simulink model "HybridControllerD2D2withRot"  (R2015b)
settings: Solver=FixedStepDiscrete  SolverMode=SingleTasking  StartTime=0.0  StopTime=inf  FixedStep=controlPeriod  RelTol=1e-3
PreLoadFcn:
  | initializeSimulation
  | initializeSCRAMNetGT
  | ATS_setup_withRot
values from neighbouring files (symbols this model uses):
  controlPeriod = 1/2048    (= 0.00048828125)    [initializeSCRAMNetGT.m]
  MRC = [2 0.05 0.001]    [ATS_setup.m]
  nAcc = 11    [initializeSCRAMNetGT.m]
  nAct = 12    [initializeSCRAMNetGT.m]
  nAdcU = 40    [initializeSCRAMNetGT.m]
  nDucU = 4    [initializeSCRAMNetGT.m]
  Nl = floor(tl*sample_rate)    [ATS_setup.m]
  node = scgtnodestruct(node)    [initializeSCRAMNetGT.m]
  nTbl = 6    [initializeSCRAMNetGT.m]
  P_range = [0.7 1.30 ... (first row only)    [ATS_setup.m]
  sample = 1/2048    (= 0.00048828125)    [ATS_setup.m]
  SN = 16    [ATS_setup.m]
  Zden = ztag.Denominator{1}    [ATS_setup.m]
  Zden_Frc = ztag_Frc.Denominator{1}    [ATS_setup.m]
  Znum = ztag.Numerator{1}    [ATS_setup.m]
  Znum_Frc = ztag_Frc.Numerator{1}    [ATS_setup.m]
undefined symbols (not defined in the file or in its folder): msc150checks
undefined symbols (not defined in the file): HybridCtrlParameters, Par, Threshold
libraries: simulink x14, slrtlib x12, cwcec_scgtLib x4
(part 1 of 2)
CloseFcn:
  | rtwprivate ssgencode ModelCloseRequest scrnet_receiver
settings Model: ExtModeArmWhenConnect=off  Creator=aschellenberg  LastModifiedBy=Andreas
settings SolverCC: EnableConcurrentExecution=on
settings DataIOCC: LimitDataPoints=off  SaveFormat=Array  SaveOutput=off  SignalLogging=off  SaveTime=off  SignalLoggingName=sigsOut
settings OptimizationCC: BlockReduction=off  OptimizeBlockIOStorage=off  BufferReuse=off  GlobalBufferReuse=off  ExpressionFolding=off  ExpressionDepthLimit=2147483647  LocalBlockOutputs=off  InitFltsAndDblsToZero=on  EfficientFloat2IntCast=on  SimCompilerOptimization=on
settings DebuggingCC: SaveWithParameterizedLinksMsg=none  CheckSSInitialOutputMsg=off  UnderspecifiedInitializationDetection=Classic  MergeDetectMultiDrivingBlocksExec=none  StateNameClashWarn=warning
settings HardwareCC: ProdBitPerPointer=32  ProdLargestAtomicFloat=None  ProdWordSize=32  ProdLongLongMode=on  ProdHWDeviceType=Generic->32-bit x86 compatible  TargetHWDeviceType=32-bit Generic
settings SFSimCC: SimCustomHeaderCode="#include \"PredictorCorrector.h\""  SimUserSources=PredictorCorrector.c  SimUserIncludeDirs="\"C:\\Program Files\\OpenFresco\\SourceCode\\SRC\\experimentalControl\\Simulink\\HybridSimToolbox\""
settings RTWCC: SystemTargetFile=slrt.tlc  TemplateMakefile=slrt_default_tmf  Description=Simulink Real-Time  CustomHeaderCode="#include \"PredictorCorrector.h\""  CustomInclude="\"C:\\Program Files\\OpenFresco\\SourceCode\\SRC\\experimentalControl\\Simulink\\HybridSimToolbox\""  CustomSource=PredictorCorrector.c  RTWCompilerOptimization=on
settings SimulinkRealTimeCC: TargetFcnLib=ansi_tfl_tmw.mat  GeneratePreprocessorConditionals=Disable all  RL32IRQSourceModifier=Auto (PCI only)  xPCIRQSourceBoard=SCRAMNet_GT200
settings ConfigComp: CovModelRefEnable=Off  CovSFcnEnable=off

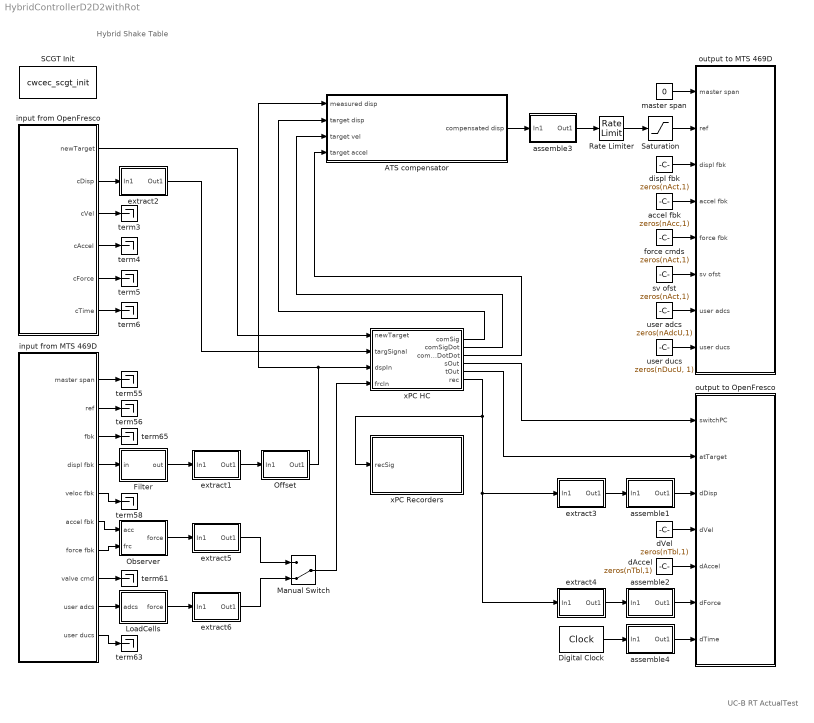
== system HybridControllerD2D2withRot ==
  note: Hybrid Shake Table
  note: UC-B RT ActualTest
  ATS compensator : Subsystem  mask{param=Par, threshold=Threshold}
      mask prompts: param "Initial a0, a1, a2 values :"; threshold "Threshold for triggering ATS :"
  Digital Clock : DigitalClock  SampleTime=controlPeriod
  Filter : Subsystem
  LoadCells : Subsystem
  Manual Switch : ManualSwitch  CurrentSetting=0
  Observer : Subsystem
  Offset : Subsystem  mask(Signal Offset){nS=HybridCtrlParameters.nDOF, nOffset=1}
      mask prompts: nS "Number of Signals: nS"; nOffset "Number of samples to initialize offset: nOffset"
      mask help:
      | Offset signal by average of signal over initial number of samples.
      | Set nOffset = -1 for no signal offset.
      mask Display: fprintf('Signal\nOffset')
  Rate Limiter : RateLimiter  RisingSlewLimit=[30 30 30 15 15 15]  FallingSlewLimit=-[30 30 30 15 15 15]  SampleTimeMode=inherited
  "SCGT Init " : S-Function  InitFcn=msc150checks(1)  FunctionName=cwcec_scgt_init  Parameters=node(1).Interface.Internal.NodeID, node(1).Interface.Internal.ActiveInterface, node.Interface.Internal.Options, node(1).Interface.Internal.Mask, pci  SFunctionDeploymentMode=off  EnableBusSupport=off  mask(SCGT Init){node=node, pci=-1}
      mask prompts: node "Node struct:"; pci "PCI slot (-1: autosearch):"
      mask help: Configures the SCRAMNet GT shared memory board. This is a required block for any model that uses shared memory with the SCRAMNet GT board. It configures important registers on the board acording to the user-defined node structure.
      mask init:
      | node=scgtnodestruct(node);
      mask Help: web([matlabroot '/toolbox/rtw/targets/xpc/target/build/xpcblocks/thirdpartydrivers/cwcec_scgthelp/'  'scgt5.html'])
      mask Display: disp('init')
  Saturation : Saturate  UpperLimit=[4.9 4.9 1.9 0.9 0.9 0.9]  LowerLimit=[-4.9 -4.9 -1.9 -0.9 -0.9 -0.9]
  accel fbk : Constant  Value=zeros(nAcc,1)
  assemble1 : Subsystem  mask(to Actuators){id=[1 2 3 4], size=nTbl}
      mask prompts: id "Index Vector: id"; size "Vector Size: size"
      mask help: To select to which actuator(s) the signals are going to
      mask Display: disp('Assemble')
  assemble2 : Subsystem  mask(to Actuators){id=[1 2 3 4], size=nTbl}
      mask prompts: id "Index Vector: id"; size "Vector Size: size"
      mask help: To select to which actuator(s) the signals are going to
      mask Display: disp('Assemble')
  assemble3 : Subsystem  mask(to Actuators){id=[1 2 4 5], size=nTbl}
      mask prompts: id "Index Vector: id"; size "Vector Size: size"
      mask help: To select to which actuator(s) the signals are going to
      mask Display: disp('Assemble')
  assemble4 : Subsystem  mask(to Actuators){id=1, size=nTbl}
      mask prompts: id "Index Vector: id"; size "Vector Size: size"
      mask help: To select to which actuator(s) the signals are going to
      mask Display: disp('Assemble')
  dAccel : Constant  Value=zeros(nTbl,1)
  dVel : Constant  Value=zeros(nTbl,1)
  displ fbk : Constant  Value=zeros(nAct,1)
  extract1 : Subsystem  mask(from Actuators){id=[1 2 4 5], size=5}
      mask prompts: id "Index Vector: id"; size "Vector Size: size"
      mask help: To select from which actuator(s) the signals are coming from
      mask Display: disp('Extract')
  extract2 : Subsystem  mask(from Actuators){id=[1 2 3 4], size=nTbl}
      mask prompts: id "Index Vector: id"; size "Vector Size: size"
      mask help: To select from which actuator(s) the signals are coming from
      mask Display: disp('Extract')
  extract3 : Subsystem  mask(from Actuators){id=[4*HybridCtrlParameters.nDOF+1:5*HybridCtrlParameters.nDOF], size=5+8*HybridCtrlParameters.nDOF}
      mask prompts: id "Index Vector: id"; size "Vector Size: size"
      mask help: To select from which actuator(s) the signals are coming from
      mask Display: disp('Extract')
  extract4 : Subsystem  mask(from Actuators){id=[5*HybridCtrlParameters.nDOF+1:6*HybridCtrlParameters.nDOF], size=5+8*HybridCtrlParameters.nDOF}
      mask prompts: id "Index Vector: id"; size "Vector Size: size"
      mask help: To select from which actuator(s) the signals are coming from
      mask Display: disp('Extract')
  extract5 : Subsystem  mask(from Actuators){id=[1 2 4 5], size=nTbl}
      mask prompts: id "Index Vector: id"; size "Vector Size: size"
      mask help: To select from which actuator(s) the signals are coming from
      mask Display: disp('Extract')
  extract6 : Subsystem  mask(from Actuators){id=[1 2 4 5], size=5}
      mask prompts: id "Index Vector: id"; size "Vector Size: size"
      mask help: To select from which actuator(s) the signals are coming from
      mask Display: disp('Extract')
  force cmds : Constant  Value=zeros(nAct,1)
  input from MTS 469D : Subsystem
  input from OpenFresco : Subsystem
  master span : Constant  Value=0
  output to MTS 469D : Subsystem
  output to OpenFresco : Subsystem
  sv ofst : Constant  Value=zeros(nAct,1)
  term{3..6,55..56,58,61,63,65} (10 alike) : Terminator
  user adcs : Constant  Value=zeros(nAdcU,1)
  user ducs : Constant  Value=zeros(nDucU, 1)  OutDataTypeStr=uint32
  xPC HC : Subsystem  mask(Hybrid Controller: D2/D2){nDOF=HybridCtrlParameters.nDOF, upFact=HybridCtrlParameters.upFact, dtInt=HybridCtrlParameters.dtInt, dtSim=HybridCtrlParameters.dtSim, dtCon=HybridCtrlParameters.dtCon, N=HybridCtrlParameters.N, iDelay=HybridCtrlParameters.iDelay}
      mask prompts: nDOF "Number of DOF: nDOF"; upFact "Upsample Factor: upFact"; dtInt "Integration time step: dtInt"; dtSim "Simulation time step: dtSim"; dtCon "Controller time step: dtCon"; N "Number of substeps: N"; iDelay "Number of delay steps: iDelay"
      mask help: Hybrid Controller using C0-continuous quadratic Lagrange interpolation for prediction and correction
      mask Display: disp('xPC Target\nHybrid Controller\n(D2/D2)')
  xPC Recorders : Subsystem  mask{nDOF=HybridCtrlParameters.nDOF}
      mask prompts: nDOF "Number of DOF: nDOF"
  wires:
  dVel/1 -> output to OpenFresco/4(dVel)
  dAccel/1 -> output to OpenFresco/5(dAccel)
  assemble4/1(Out1) -> output to OpenFresco/7(dTime)
  input from OpenFresco/3(cVel) -> term3/1
  input from OpenFresco/5(cForce) -> term5/1
  input from OpenFresco/6(cTime) -> term6/1
  assemble1/1(Out1) -> output to OpenFresco/3(dDisp)
  assemble2/1(Out1) -> output to OpenFresco/6(dForce)
  input from OpenFresco/2(cDisp) -> extract2/1(In1)
  input from OpenFresco/4(cAccel) -> term4/1
  input from OpenFresco/1(newTarget) -> xPC HC/1(newTarget)
  xPC HC/4(sOut) -> output to OpenFresco/1(switchPC)
  xPC HC/5(tOut) -> output to OpenFresco/2(atTarget)
  extract3/1(Out1) -> assemble1/1(In1)
  extract4/1(Out1) -> assemble2/1(In1)
  master span/1 -> output to MTS 469D/1(master span)
  force cmds/1 -> output to MTS 469D/5(force fbk)
  displ fbk/1 -> output to MTS 469D/3(displ fbk)
  user ducs/1 -> output to MTS 469D/8(user ducs)
  accel fbk/1 -> output to MTS 469D/4(accel fbk)
  user adcs/1 -> output to MTS 469D/7(user adcs)
  sv ofst/1 -> output to MTS 469D/6(sv ofst)
  Saturation/1 -> output to MTS 469D/2(ref)
  extract1/1(Out1) -> Offset/1(In1)
  input from MTS 469D/10(user ducs) -> term63/1
  input from MTS 469D/9(user adcs) -> LoadCells/1(adcs)
  input from MTS 469D/8(valve cmd) -> term61/1
  input from MTS 469D/7(force fbk) -> Observer/2(frc)
  input from MTS 469D/6(accel fbk) -> Observer/1(acc)
  input from MTS 469D/5(veloc fbk) -> term58/1
  input from MTS 469D/4(displ fbk) -> Filter/1(in)
  input from MTS 469D/2(ref) -> term56/1
  input from MTS 469D/1(master span) -> term55/1
  input from MTS 469D/3(fbk) -> term65/1
  Observer/1(force) -> extract5/1(In1)
  LoadCells/1(force) -> extract6/1(In1)
  xPC HC/6(rec) -> extract3/1(In1), extract4/1(In1), xPC Recorders/1(recSig)
  extract5/1(Out1) -> Manual Switch/1
  extract6/1(Out1) -> Manual Switch/2
  xPC HC/1(comSig) -> ATS compensator/2(target disp)
  xPC HC/2(comSigDot) -> ATS compensator/3(target vel)
  xPC HC/3(comSigDotDot) -> ATS compensator/4(target accel)
  Digital Clock/1 -> assemble4/1(In1)
  extract2/1(Out1) -> xPC HC/2(targSignal)
  Manual Switch/1 -> xPC HC/4(frcIn)
  Offset/1(Out1) -> ATS compensator/1(measured disp), xPC HC/3(dspIn)
  Filter/1(out) -> extract1/1(In1)
  Rate Limiter/1 -> Saturation/1
  ATS compensator/1(compensated disp) -> assemble3/1(In1)
  assemble3/1(Out1) -> Rate Limiter/1

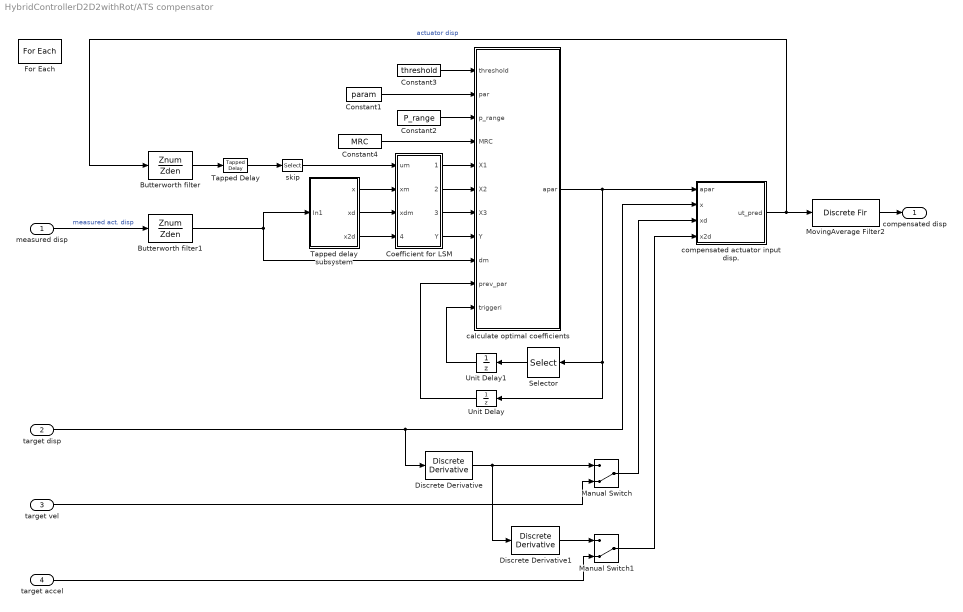
== system HybridControllerD2D2withRot/ATS compensator ==
  measured disp : Inport  Partition=on  PartitionDimension=1  PartitionWidth=1
  target disp : Inport  Port=2  Partition=on  PartitionDimension=1  PartitionWidth=1
  target vel : Inport  Port=3  Partition=on  PartitionDimension=1  PartitionWidth=1
  target accel : Inport  Port=4  Partition=on  PartitionDimension=1  PartitionWidth=1
  Butterworth filter : DiscreteTransferFcn  Numerator=Znum  Denominator=Zden  SampleTime=sample
  Butterworth filter1 : DiscreteTransferFcn  Numerator=Znum  Denominator=Zden  SampleTime=sample
  Coefficient for LSM : Subsystem
  Constant1 : Constant  Value=param
  Constant2 : Constant  Value=P_range
  Constant3 : Constant  Value=threshold
  Constant4 : Constant  Value=MRC
  Discrete Derivative : simulink/Discrete/Discrete Derivative  gainval=1.0  ICPrevScaledInput=0.0  OutMin=[]  OutMax=[]  OutDataType=fixdt(1, 16)  OutScaling=2^-10  DoSatur=off
  Discrete Derivative1 : simulink/Discrete/Discrete Derivative  gainval=1.0  ICPrevScaledInput=0.0  OutMin=[]  OutMax=[]  OutDataType=fixdt(1, 16)  OutScaling=2^-10  DoSatur=off
  For Each : ForEach  DisableCoverage=on  IterateSubsysMaskParameter=on,on  SubsysMaskParameterIterationDimension=2,2  IndexMode=One-based
  Manual Switch : ManualSwitch  CurrentSetting=0
  Manual Switch1 : ManualSwitch  CurrentSetting=0
  MovingAverage Filter2 : DiscreteFir  Coefficients=1/numSample*ones(1,numSample)  mask(Moving Average Filter){numSample=10}
      mask prompts: numSample "Number of Samples: numSample"
      mask help:
      | Moving average filter by using discrete FIR filter.
      | Set numSample = 1 for no filtering.
      mask Display: fprintf('MovingAverage\nFilter')
  Selector : Selector  InputPortWidth=4  IndexOptions=Index vector (dialog)  Indices=4  OutputSizes=1
  Tapped Delay : simulink/Discrete/Tapped Delay  vinit=0.0  samptime=-1  NumDelays=Nl  DelayOrder=Oldest  includeCurrent=off
  Tapped delay subsystem : Subsystem
  Unit Delay : UnitDelay  SampleTime=-1
  Unit Delay1 : UnitDelay  SampleTime=-1
  calculate optimal coefficients : MATLAB Function  TreatAsAtomicUnit=on
  compensated actuator input disp. : MATLAB Function  TreatAsAtomicUnit=on
  skip : Selector  InputPortWidth=Nl  IndexOptions=Index vector (dialog)  Indices=[1:SN:Nl]  OutputSizes=1
  compensated disp : Outport  ConcatenationDimension=1
  wires:
  measured disp/1 -> Butterworth filter1/1  "measured act. disp"
  Tapped Delay/1 -> skip/1
  calculate optimal coefficients/1(apar) -> Unit Delay/1, Selector/1, compensated actuator input disp./1(apar)
  compensated actuator input disp./1(ut_pred) -> MovingAverage Filter2/1, Butterworth filter/1  "actuator disp"
  Constant1/1 -> calculate optimal coefficients/2(par)
  Constant2/1 -> calculate optimal coefficients/3(p_range)
  Unit Delay/1 -> calculate optimal coefficients/10(prev_par)
  target disp/1 -> compensated actuator input disp./2(x), Discrete Derivative/1
  skip/1 -> Coefficient for LSM/1(um)
  Tapped delay subsystem/1(x) -> Coefficient for LSM/2(xm)
  Tapped delay subsystem/2(xd) -> Coefficient for LSM/3(xdm)
  Tapped delay subsystem/3(x2d) -> Coefficient for LSM/4(x2dm)
  Coefficient for LSM/1(X(1,:)) -> calculate optimal coefficients/5(X1)
  Coefficient for LSM/2(X(2,:)) -> calculate optimal coefficients/6(X2)
  Coefficient for LSM/3(X(3,:)) -> calculate optimal coefficients/7(X3)
  Coefficient for LSM/4(Y) -> calculate optimal coefficients/8(Y)
  Unit Delay1/1 -> calculate optimal coefficients/11(triggeri)
  Constant3/1 -> calculate optimal coefficients/1(threshold)
  Butterworth filter/1 -> Tapped Delay/1
  Constant4/1 -> calculate optimal coefficients/4(MRC)
  Selector/1 -> Unit Delay1/1
  Manual Switch/1 -> compensated actuator input disp./3(xd)
  Discrete Derivative/1 -> Manual Switch/1, Discrete Derivative1/1
  target vel/1 -> Manual Switch/2
  Discrete Derivative1/1 -> Manual Switch1/1
  Manual Switch1/1 -> compensated actuator input disp./4(x2d)
  target accel/1 -> Manual Switch1/2
  Butterworth filter1/1 -> Tapped delay subsystem/1(In1), calculate optimal coefficients/9(dm)
  MovingAverage Filter2/1 -> compensated disp/1

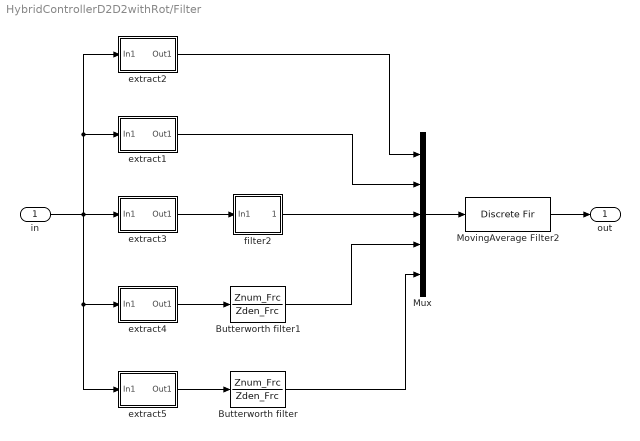
== system HybridControllerD2D2withRot/Filter ==
  in : Inport
  Butterworth filter : DiscreteTransferFcn  Numerator=Znum_Frc  Denominator=Zden_Frc  SampleTime=controlPeriod
  Butterworth filter1 : DiscreteTransferFcn  Numerator=Znum_Frc  Denominator=Zden_Frc  SampleTime=controlPeriod
  MovingAverage Filter2 : DiscreteFir  Coefficients=1/numSample*ones(1,numSample)  mask(Moving Average Filter){numSample=10}
      mask prompts: numSample "Number of Samples: numSample"
      mask help:
      | Moving average filter by using discrete FIR filter.
      | Set numSample = 1 for no filtering.
      mask Display: fprintf('MovingAverage\nFilter')
  Mux : Mux  Inputs=5
  extract1 : Subsystem  mask(from Actuators){id=2, size=nTbl}
      mask prompts: id "Index Vector: id"; size "Vector Size: size"
      mask help: To select from which actuator(s) the signals are coming from
      mask Display: disp('Extract')
  extract2 : Subsystem  mask(from Actuators){id=1, size=nTbl}
      mask prompts: id "Index Vector: id"; size "Vector Size: size"
      mask help: To select from which actuator(s) the signals are coming from
      mask Display: disp('Extract')
  extract3 : Subsystem  mask(from Actuators){id=3, size=nTbl}
      mask prompts: id "Index Vector: id"; size "Vector Size: size"
      mask help: To select from which actuator(s) the signals are coming from
      mask Display: disp('Extract')
  extract4 : Subsystem  mask(from Actuators){id=4, size=nTbl}
      mask prompts: id "Index Vector: id"; size "Vector Size: size"
      mask help: To select from which actuator(s) the signals are coming from
      mask Display: disp('Extract')
  extract5 : Subsystem  mask(from Actuators){id=5, size=nTbl}
      mask prompts: id "Index Vector: id"; size "Vector Size: size"
      mask help: To select from which actuator(s) the signals are coming from
      mask Display: disp('Extract')
  filter2 : Subsystem
  out : Outport
  wires:
  in/1 -> extract2/1(In1), extract1/1(In1), extract5/1(In1), extract4/1(In1), extract3/1(In1)
  Mux/1 -> MovingAverage Filter2/1
  extract1/1(Out1) -> Mux/2
  filter2/1(Out1) -> Mux/3
  extract3/1(Out1) -> filter2/1(In1)
  extract2/1(Out1) -> Mux/1
  extract4/1(Out1) -> Butterworth filter1/1
  MovingAverage Filter2/1 -> out/1
  extract5/1(Out1) -> Butterworth filter/1
  Butterworth filter/1 -> Mux/5
  Butterworth filter1/1 -> Mux/4

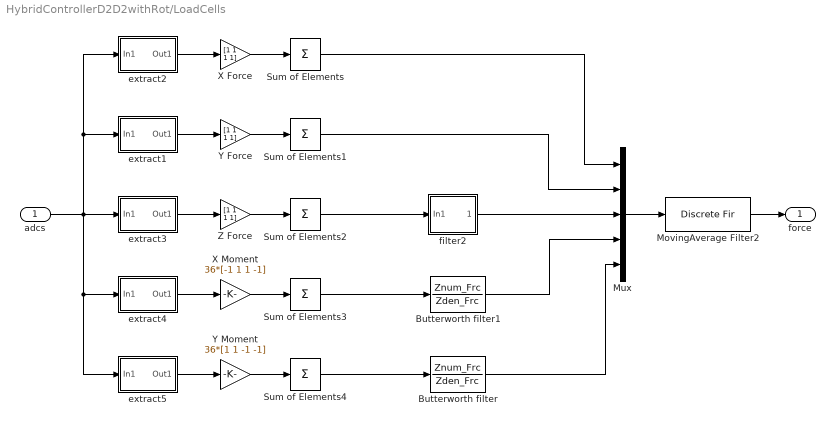
== system HybridControllerD2D2withRot/LoadCells ==
  adcs : Inport
  Butterworth filter : DiscreteTransferFcn  Numerator=Znum_Frc  Denominator=Zden_Frc  SampleTime=controlPeriod
  Butterworth filter1 : DiscreteTransferFcn  Numerator=Znum_Frc  Denominator=Zden_Frc  SampleTime=controlPeriod
  MovingAverage Filter2 : DiscreteFir  Coefficients=1/numSample*ones(1,numSample)  mask(Moving Average Filter){numSample=10}
      mask prompts: numSample "Number of Samples: numSample"
      mask help:
      | Moving average filter by using discrete FIR filter.
      | Set numSample = 1 for no filtering.
      mask Display: fprintf('MovingAverage\nFilter')
  Mux : Mux  Inputs=5
  Sum of Elements{,1..4} (5 alike) : Sum  Inputs=+
  X Force : Gain  Gain=[1 1 1 1]
  X Moment : Gain  Gain=36*[-1 1 1 -1]
  Y Force : Gain  Gain=[1 1 1 1]
  Y Moment : Gain  Gain=36*[1 1 -1 -1]
  Z Force : Gain  Gain=[1 1 1 1]
  extract1 : Subsystem  mask(from Actuators){id=[3 8 13 18], size=nAdcU}
      mask prompts: id "Index Vector: id"; size "Vector Size: size"
      mask help: To select from which actuator(s) the signals are coming from
      mask Display: disp('Extract')
  extract2 : Subsystem  mask(from Actuators){id=[2 7 12 17], size=nAdcU}
      mask prompts: id "Index Vector: id"; size "Vector Size: size"
      mask help: To select from which actuator(s) the signals are coming from
      mask Display: disp('Extract')
  extract3 : Subsystem  mask(from Actuators){id=[1 6 11 16], size=nAdcU}
      mask prompts: id "Index Vector: id"; size "Vector Size: size"
      mask help: To select from which actuator(s) the signals are coming from
      mask Display: disp('Extract')
  extract4 : Subsystem  mask(from Actuators){id=[1 6 11 16], size=nAdcU}
      mask prompts: id "Index Vector: id"; size "Vector Size: size"
      mask help: To select from which actuator(s) the signals are coming from
      mask Display: disp('Extract')
  extract5 : Subsystem  mask(from Actuators){id=[1 6 11 16], size=nAdcU}
      mask prompts: id "Index Vector: id"; size "Vector Size: size"
      mask help: To select from which actuator(s) the signals are coming from
      mask Display: disp('Extract')
  filter2 : Subsystem
  force : Outport
  wires:
  extract2/1(Out1) -> X Force/1
  adcs/1 -> extract2/1(In1), extract1/1(In1), extract5/1(In1), extract4/1(In1), extract3/1(In1)
  X Force/1 -> Sum of Elements/1
  extract1/1(Out1) -> Y Force/1
  Y Force/1 -> Sum of Elements1/1
  extract3/1(Out1) -> Z Force/1
  Z Force/1 -> Sum of Elements2/1
  Mux/1 -> MovingAverage Filter2/1
  Sum of Elements1/1 -> Mux/2
  Sum of Elements2/1 -> filter2/1(In1)
  filter2/1(Out1) -> Mux/3
  Sum of Elements/1 -> Mux/1
  extract4/1(Out1) -> X Moment/1
  X Moment/1 -> Sum of Elements3/1
  Sum of Elements3/1 -> Butterworth filter1/1
  extract5/1(Out1) -> Y Moment/1
  Y Moment/1 -> Sum of Elements4/1
  MovingAverage Filter2/1 -> force/1
  Sum of Elements4/1 -> Butterworth filter/1
  Butterworth filter/1 -> Mux/5
  Butterworth filter1/1 -> Mux/4

== system HybridControllerD2D2withRot/Observer ==
  acc : Inport
  frc : Inport  Port=2
  Add : Sum  Inputs=-+
  Mtable : Gain  Gain=[86.8 86.8 86.8 0.0 0.0 0.0]
  force : Outport
  wires:
  acc/1 -> Mtable/1
  Mtable/1 -> Add/1
  frc/1 -> Add/2
  Add/1 -> force/1

== system HybridControllerD2D2withRot/Offset ==
  In1 : Inport
  Constant : Constant  Value=zeros(1,nS)
  Counter : simulink/Sources/Counter Free-Running  NumBits=32  tsamp=controlPeriod
  Data Store Memory : DataStoreMemory  DataStoreName=x0  InitialValue=zeros(1,nS)  OutDataTypeStr=double
  Data Store Read : DataStoreRead  DataStoreName=x0  SampleTime=controlPeriod
  If : If  IfExpression=u1 < nOffset  ShowElse=off
  If Action : Subsystem  TreatAsAtomicUnit=on
  Sum1 : Sum  Inputs=+-|  SaturateOnIntegerOverflow=on  InputSameDT=on  OutDataTypeStr=Inherit: Same as first input
  Switch : Switch  Threshold=nOffset  SaturateOnIntegerOverflow=on  InputSameDT=on
  typeConv12 : DataTypeConversion  OutDataTypeStr=double  SaturateOnIntegerOverflow=on  RndMeth=Zero
  Out1 : Outport
  wires:
  Switch/1 -> Out1/1
  Sum1/1 -> Switch/1
  Data Store Read/1 -> Sum1/2
  In1/1 -> If Action/1(In1), Sum1/1
  Constant/1 -> Switch/3
  Counter/1 -> typeConv12/1
  If/1 -> If Action/Action
  typeConv12/1 -> Switch/2, If/1

== system HybridControllerD2D2withRot/assemble1 ==
  In1 : Inport
  Assignment : Assignment  OutputInitialize=Specify size for each dimension in table  IndexOptions=Index vector (port)  Indices=1  OutputSizes=size
  Constant : Constant  Value=id
  Out1 : Outport
  wires:
  Constant/1 -> Assignment/2
  Assignment/1 -> Out1/1
  In1/1 -> Assignment/1

== system HybridControllerD2D2withRot/assemble2 ==
  In1 : Inport
  Assignment : Assignment  OutputInitialize=Specify size for each dimension in table  IndexOptions=Index vector (port)  Indices=1  OutputSizes=size
  Constant : Constant  Value=id
  Out1 : Outport
  wires:
  Constant/1 -> Assignment/2
  Assignment/1 -> Out1/1
  In1/1 -> Assignment/1

== system HybridControllerD2D2withRot/assemble3 ==
  In1 : Inport
  Assignment : Assignment  OutputInitialize=Specify size for each dimension in table  IndexOptions=Index vector (port)  Indices=1  OutputSizes=size
  Constant : Constant  Value=id
  Out1 : Outport
  wires:
  Constant/1 -> Assignment/2
  Assignment/1 -> Out1/1
  In1/1 -> Assignment/1

== system HybridControllerD2D2withRot/assemble4 ==
  In1 : Inport
  Assignment : Assignment  OutputInitialize=Specify size for each dimension in table  IndexOptions=Index vector (port)  Indices=1  OutputSizes=size
  Constant : Constant  Value=id
  Out1 : Outport
  wires:
  Constant/1 -> Assignment/2
  Assignment/1 -> Out1/1
  In1/1 -> Assignment/1

== system HybridControllerD2D2withRot/extract1 ==
  In1 : Inport
  Selector : Selector  InputPortWidth=size  IndexOptions=Index vector (dialog)  Indices=id  OutputSizes=1
  Out1 : Outport
  wires:
  Selector/1 -> Out1/1
  In1/1 -> Selector/1

== system HybridControllerD2D2withRot/extract2 ==
  In1 : Inport
  Selector : Selector  InputPortWidth=size  IndexOptions=Index vector (dialog)  Indices=id  OutputSizes=1
  Out1 : Outport
  wires:
  Selector/1 -> Out1/1
  In1/1 -> Selector/1

== system HybridControllerD2D2withRot/extract3 ==
  In1 : Inport
  Selector : Selector  InputPortWidth=size  IndexOptions=Index vector (dialog)  Indices=id  OutputSizes=1
  Out1 : Outport
  wires:
  Selector/1 -> Out1/1
  In1/1 -> Selector/1

== system HybridControllerD2D2withRot/extract4 ==
  In1 : Inport
  Selector : Selector  InputPortWidth=size  IndexOptions=Index vector (dialog)  Indices=id  OutputSizes=1
  Out1 : Outport
  wires:
  Selector/1 -> Out1/1
  In1/1 -> Selector/1

== system HybridControllerD2D2withRot/extract5 ==
  In1 : Inport
  Selector : Selector  InputPortWidth=size  IndexOptions=Index vector (dialog)  Indices=id  OutputSizes=1
  Out1 : Outport
  wires:
  Selector/1 -> Out1/1
  In1/1 -> Selector/1

== system HybridControllerD2D2withRot/extract6 ==
  In1 : Inport
  Selector : Selector  InputPortWidth=size  IndexOptions=Index vector (dialog)  Indices=id  OutputSizes=1
  Out1 : Outport
  wires:
  Selector/1 -> Out1/1
  In1/1 -> Selector/1

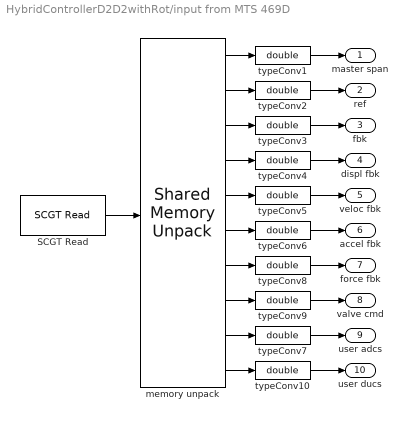
== system HybridControllerD2D2withRot/input from MTS 469D ==
  "SCGT Read " : cwcec_scgtLib/SCGT Read   partition=node.Partitions(9:18)  ts=controlPeriod  pci=-1
  memory unpack : slrtlib/Shared Memory/Shared Memory Unpack   partition=node.Partitions(9:18)
  typeConv{1..10} (10 alike) : DataTypeConversion  OutDataTypeStr=double  SaturateOnIntegerOverflow=on  RndMeth=Zero
  master span : Outport
  ref : Outport  Port=2
  fbk : Outport  Port=3
  displ fbk : Outport  Port=4
  veloc fbk : Outport  Port=5
  accel fbk : Outport  Port=6
  force fbk : Outport  Port=7
  valve cmd : Outport  Port=8
  user adcs : Outport  Port=9
  user ducs : Outport  Port=10
  wires:
  memory unpack/10 -> typeConv10/1
  memory unpack/9 -> typeConv7/1
  memory unpack/8 -> typeConv9/1
  memory unpack/7 -> typeConv8/1
  memory unpack/6 -> typeConv6/1
  memory unpack/5 -> typeConv5/1
  memory unpack/4 -> typeConv4/1
  memory unpack/3 -> typeConv3/1
  memory unpack/2 -> typeConv2/1
  memory unpack/1 -> typeConv1/1
  typeConv2/1 -> ref/1
  typeConv1/1 -> master span/1
  "SCGT Read "/1 -> memory unpack/1
  typeConv3/1 -> fbk/1
  typeConv4/1 -> displ fbk/1
  typeConv5/1 -> veloc fbk/1
  typeConv6/1 -> accel fbk/1
  typeConv8/1 -> force fbk/1
  typeConv9/1 -> valve cmd/1
  typeConv7/1 -> user adcs/1
  typeConv10/1 -> user ducs/1

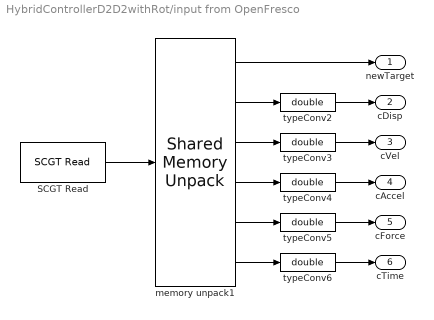
== system HybridControllerD2D2withRot/input from OpenFresco ==
  SCGT Read : cwcec_scgtLib/SCGT Read   partition=node.Partitions(19:24)  ts=controlPeriod  pci=-1
  memory unpack1 : slrtlib/Shared Memory/Shared Memory Unpack   partition=node.Partitions(19:24)
  typeConv{2..6} (5 alike) : DataTypeConversion  OutDataTypeStr=double  SaturateOnIntegerOverflow=on  RndMeth=Zero
  newTarget : Outport
  cDisp : Outport  Port=2
  cVel : Outport  Port=3
  cAccel : Outport  Port=4
  cForce : Outport  Port=5
  cTime : Outport  Port=6
  wires:
  typeConv2/1 -> cDisp/1
  typeConv3/1 -> cVel/1
  typeConv4/1 -> cAccel/1
  typeConv5/1 -> cForce/1
  typeConv6/1 -> cTime/1
  memory unpack1/3 -> typeConv3/1
  memory unpack1/4 -> typeConv4/1
  memory unpack1/6 -> typeConv6/1
  memory unpack1/5 -> typeConv5/1
  SCGT Read/1 -> memory unpack1/1
  memory unpack1/2 -> typeConv2/1
  memory unpack1/1 -> newTarget/1

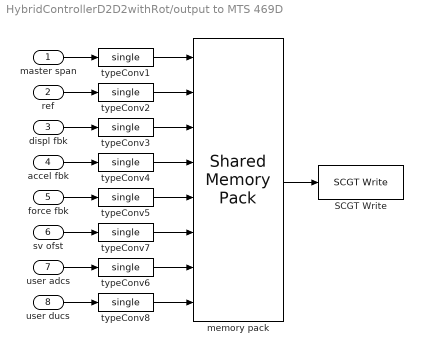
== system HybridControllerD2D2withRot/output to MTS 469D ==
  master span : Inport
  ref : Inport  Port=2
  displ fbk : Inport  Port=3
  accel fbk : Inport  Port=4
  force fbk : Inport  Port=5
  sv ofst : Inport  Port=6
  user adcs : Inport  Port=7
  user ducs : Inport  Port=8
  "SCGT Write " : cwcec_scgtLib/SCGT Write   partition=node.Partitions(1:8)  ts=controlPeriod  pci=-1
  memory pack : slrtlib/Shared Memory/Shared Memory Pack   partition=node.Partitions(1:8)
  typeConv{1..8} (8 alike) : DataTypeConversion  OutDataTypeStr=single  SaturateOnIntegerOverflow=on  RndMeth=Zero
  wires:
  typeConv8/1 -> memory pack/8
  user ducs/1 -> typeConv8/1
  user adcs/1 -> typeConv6/1
  sv ofst/1 -> typeConv7/1
  master span/1 -> typeConv1/1
  ref/1 -> typeConv2/1
  displ fbk/1 -> typeConv3/1
  accel fbk/1 -> typeConv4/1
  memory pack/1 -> "SCGT Write "/1
  typeConv1/1 -> memory pack/1
  typeConv2/1 -> memory pack/2
  typeConv3/1 -> memory pack/3
  typeConv4/1 -> memory pack/4
  force fbk/1 -> typeConv5/1
  typeConv5/1 -> memory pack/5
  typeConv7/1 -> memory pack/6
  typeConv6/1 -> memory pack/7

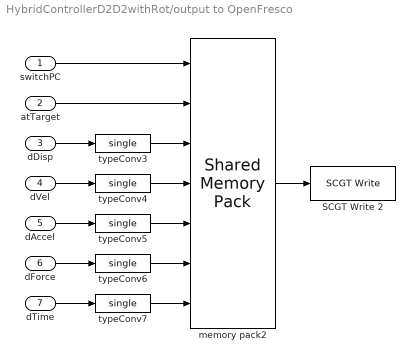
== system HybridControllerD2D2withRot/output to OpenFresco ==
  switchPC : Inport
  atTarget : Inport  Port=2
  dDisp : Inport  Port=3
  dVel : Inport  Port=4
  dAccel : Inport  Port=5
  dForce : Inport  Port=6
  dTime : Inport  Port=7
  SCGT Write 2 : cwcec_scgtLib/SCGT Write   partition=node.Partitions(25:31)  ts=controlPeriod  pci=-1
  memory pack2 : slrtlib/Shared Memory/Shared Memory Pack   partition=node.Partitions(25:31)
  typeConv{3..7} (5 alike) : DataTypeConversion  OutDataTypeStr=single  SaturateOnIntegerOverflow=on  RndMeth=Zero
  wires:
  dAccel/1 -> typeConv5/1
  dVel/1 -> typeConv4/1
  dDisp/1 -> typeConv3/1
  typeConv4/1 -> memory pack2/4
  typeConv5/1 -> memory pack2/5
  dForce/1 -> typeConv6/1
  typeConv6/1 -> memory pack2/6
  dTime/1 -> typeConv7/1
  typeConv7/1 -> memory pack2/7
  memory pack2/1 -> SCGT Write 2/1
  typeConv3/1 -> memory pack2/3
  atTarget/1 -> memory pack2/2
  switchPC/1 -> memory pack2/1

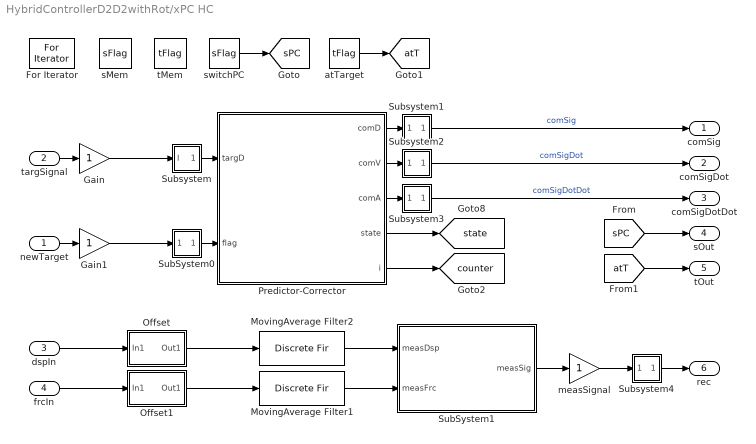
== system HybridControllerD2D2withRot/xPC HC ==
  newTarget : Inport
  targSignal : Inport  Port=2
  dspIn : Inport  Port=3
  frcIn : Inport  Port=4
  For Iterator : ForIterator  IterationLimit=upFact  ShowIterationPort=off
  Gain : Gain  OutDataTypeStr=double
  Gain1 : Gain  OutDataTypeStr=int32
  MovingAverage Filter1 : DiscreteFir  Coefficients=1/numSample*ones(1,numSample)  mask(Moving Average Filter){numSample=1}
      mask prompts: numSample "Number of Samples: numSample"
      mask help:
      | Moving average filter by using discrete FIR filter.
      | Set numSample = 1 for no filtering.
      mask Display: fprintf('MovingAverage\nFilter')
  MovingAverage Filter2 : DiscreteFir  Coefficients=1/numSample*ones(1,numSample)  mask(Moving Average Filter){numSample=1}
      mask prompts: numSample "Number of Samples: numSample"
      mask help:
      | Moving average filter by using discrete FIR filter.
      | Set numSample = 1 for no filtering.
      mask Display: fprintf('MovingAverage\nFilter')
  Offset : Subsystem  mask(Signal Offset){nS=nDOF, nOffset=1/dtCon}
      mask prompts: nS "Number of Signals: nS"; nOffset "Number of samples to initialize offset: nOffset"
      mask help:
      | Offset signal by average of signal over initial number of samples.
      | Set nOffset = -1 for no signal offset.
      mask Display: fprintf('Signal\nOffset')
  Offset1 : Subsystem  mask(Signal Offset){nS=nDOF, nOffset=1/dtCon}
      mask prompts: nS "Number of Signals: nS"; nOffset "Number of samples to initialize offset: nOffset"
      mask help:
      | Offset signal by average of signal over initial number of samples.
      | Set nOffset = -1 for no signal offset.
      mask Display: fprintf('Signal\nOffset')
  Predictor-Corrector : Stateflow chart  TreatAsAtomicUnit=on
  SubSystem0 : Subsystem
      mask Display: disp('I/O')
  SubSystem1 : Subsystem
  Subsystem : Subsystem
      mask Display: disp('I/O')
  Subsystem1 : Subsystem
      mask Display: disp('I/O')
  Subsystem2 : Subsystem
      mask Display: disp('I/O')
  Subsystem3 : Subsystem
      mask Display: disp('I/O')
  Subsystem4 : Subsystem
      mask Display: disp('I/O')
  atTarget : DataStoreRead  DataStoreName=tFlag
  measSignal : Gain  OutDataTypeStr=double
  sMem : DataStoreMemory  DataStoreName=sFlag  OutDataTypeStr=int32
  switchPC : DataStoreRead  DataStoreName=sFlag
  tMem : DataStoreMemory  DataStoreName=tFlag  OutDataTypeStr=int32
  comSig : Outport
  comSigDot : Outport  Port=2
  comSigDotDot : Outport  Port=3
  sOut : Outport  Port=4
  tOut : Outport  Port=5
  rec : Outport  Port=6
  tag scope: atT=global, counter=global, sPC=global, state=global
  wires:
  frcIn/1 -> Offset1/1(In1)
  measSignal/1 -> Subsystem4/1(measSig)
  dspIn/1 -> Offset/1(In1)
  SubSystem1/1(measSig) -> measSignal/1
  Predictor-Corrector/5(i) -> [counter]
  SubSystem0/1(Out) -> Predictor-Corrector/2(flag)
  newTarget/1 -> Gain1/1
  switchPC/1 -> [sPC]
  atTarget/1 -> [atT]
  targSignal/1 -> Gain/1
  Subsystem/1(O) -> Predictor-Corrector/1(targD)
  MovingAverage Filter2/1 -> SubSystem1/1(measDsp)
  MovingAverage Filter1/1 -> SubSystem1/2(measFrc)
  Predictor-Corrector/1(comD) -> Subsystem1/1(In)
  Predictor-Corrector/2(comV) -> Subsystem2/1(In)
  Predictor-Corrector/3(comA) -> Subsystem3/1(In)
  Gain/1 -> Subsystem/1(I)
  Gain1/1 -> SubSystem0/1(In)
  Offset/1(Out1) -> MovingAverage Filter2/1
  Predictor-Corrector/4(state) -> [state]
  Subsystem2/1(Out) -> comSigDot/1  "comSigDot"
  Subsystem3/1(Out) -> comSigDotDot/1  "comSigDotDot"
  Subsystem1/1(Out) -> comSig/1  "comSig"
  Subsystem4/1(Out1) -> rec/1
  [sPC] -> sOut/1
  [atT] -> tOut/1
  Offset1/1(Out1) -> MovingAverage Filter1/1

== system HybridControllerD2D2withRot/xPC Recorders ==
  recSig : Inport
  Demux : Demux  Outputs=[nDOF (3*nDOF) (2*nDOF) 1 1 3 nDOF nDOF]
  "Scope (xPC) " : slrtlib/Displays and Logging/Scope   scopeno=4  scopetype=File  autostart=on  viewmode=Graphical redraw  formatstr='%15.6f'  grid=on  ylimits=[0,3]  nosamples=60*2048  noprepostsamples=0  interleave=1  triggermode=FreeRun  triggersignal=1  trigsignalfromport=off  triggerlevel=0.0  triggerslope=Either  triggerscope=1  triggersample=0  filename=state.dat  mode=Lazy  writesize=512  autorestart=on  dynamicfilemode=off  maxwritefilesize=512*1024^2
  Scope (xPC) 1 : slrtlib/Displays and Logging/Scope   scopeno=1  scopetype=File  autostart=on  viewmode=Numerical  formatstr='%15.6f'  grid=on  ylimits=[-4,4]  nosamples=60*2048  noprepostsamples=0  interleave=1  triggermode=FreeRun  triggersignal=1  trigsignalfromport=off  triggerlevel=0.0  triggerslope=Either  triggerscope=1  triggersample=0  filename=targSig.dat  mode=Lazy  writesize=512  autorestart=on  dynamicfilemode=off  maxwritefilesize=512*1024^2
  Scope (xPC) 2 : slrtlib/Displays and Logging/Scope   scopeno=5  scopetype=File  autostart=on  viewmode=Numerical  formatstr='%15.6f'  grid=on  ylimits=[0,3]  nosamples=60*2048  noprepostsamples=0  interleave=1  triggermode=FreeRun  triggersignal=1  trigsignalfromport=off  triggerlevel=0.0  triggerslope=Either  triggerscope=1  triggersample=0  filename=count.dat  mode=Lazy  writesize=512  autorestart=on  dynamicfilemode=off  maxwritefilesize=512*1024^2
  Scope (xPC) 3 : slrtlib/Displays and Logging/Scope   scopeno=6  scopetype=File  autostart=on  viewmode=Numerical  formatstr='%15.6f'  grid=on  ylimits=[0,3]  nosamples=60*2048  noprepostsamples=0  interleave=1  triggermode=FreeRun  triggersignal=1  trigsignalfromport=off  triggerlevel=0.0  triggerslope=Either  triggerscope=1  triggersample=0  filename=flag.dat  mode=Lazy  writesize=512  autorestart=on  dynamicfilemode=off  maxwritefilesize=512*1024^2
  Scope (xPC) 4 : slrtlib/Displays and Logging/Scope   scopeno=2  scopetype=File  autostart=on  viewmode=Numerical  formatstr='%15.6f'  grid=on  ylimits=[-4,4]  nosamples=60*2048  noprepostsamples=0  interleave=1  triggermode=FreeRun  triggersignal=1  trigsignalfromport=off  triggerlevel=0.0  triggerslope=Either  triggerscope=1  triggersample=0  filename=commSig.dat  mode=Lazy  writesize=512  autorestart=on  dynamicfilemode=off  maxwritefilesize=512*1024^2
  Scope (xPC) 5 : slrtlib/Displays and Logging/Scope   scopeno=3  scopetype=File  autostart=on  viewmode=Numerical  formatstr='%15.6f'  grid=on  ylimits=[-4,4]  nosamples=60*2048  noprepostsamples=0  interleave=1  triggermode=FreeRun  triggersignal=1  trigsignalfromport=off  triggerlevel=0.0  triggerslope=Either  triggerscope=1  triggersample=0  filename=measSig.dat  mode=Lazy  writesize=512  autorestart=on  dynamicfilemode=off  maxwritefilesize=512*1024^2
  Scope (xPC) 6 : slrtlib/Displays and Logging/Scope   scopeno=7  scopetype=File  autostart=on  viewmode=Graphical redraw  formatstr='%15.6f'  grid=on  ylimits=[-1,1]  nosamples=60*2048  noprepostsamples=0  interleave=1  triggermode=FreeRun  triggersignal=1  trigsignalfromport=off  triggerlevel=0.0  triggerslope=Either  triggerscope=1  triggersample=0  filename=measDsp.dat  mode=Lazy  writesize=512  autorestart=on  dynamicfilemode=off  maxwritefilesize=512*1024^2
  Scope (xPC) 7 : slrtlib/Displays and Logging/Scope   scopeno=8  scopetype=File  autostart=on  viewmode=Numerical  formatstr='%15.6f'  grid=on  ylimits=[0,3]  nosamples=60*2048  noprepostsamples=0  interleave=1  triggermode=FreeRun  triggersignal=1  trigsignalfromport=off  triggerlevel=0.0  triggerslope=Either  triggerscope=1  triggersample=0  filename=measFrc.dat  mode=Lazy  writesize=512  autorestart=on  dynamicfilemode=off  maxwritefilesize=512*1024^2
  wires:
  recSig/1 -> Demux/1
  Demux/1 -> Scope (xPC) 1/1
  Demux/2 -> Scope (xPC) 4/1
  Demux/3 -> Scope (xPC) 5/1
  Demux/4 -> "Scope (xPC) "/1
  Demux/5 -> Scope (xPC) 2/1
  Demux/6 -> Scope (xPC) 3/1
  Demux/8 -> Scope (xPC) 7/1
  Demux/7 -> Scope (xPC) 6/1

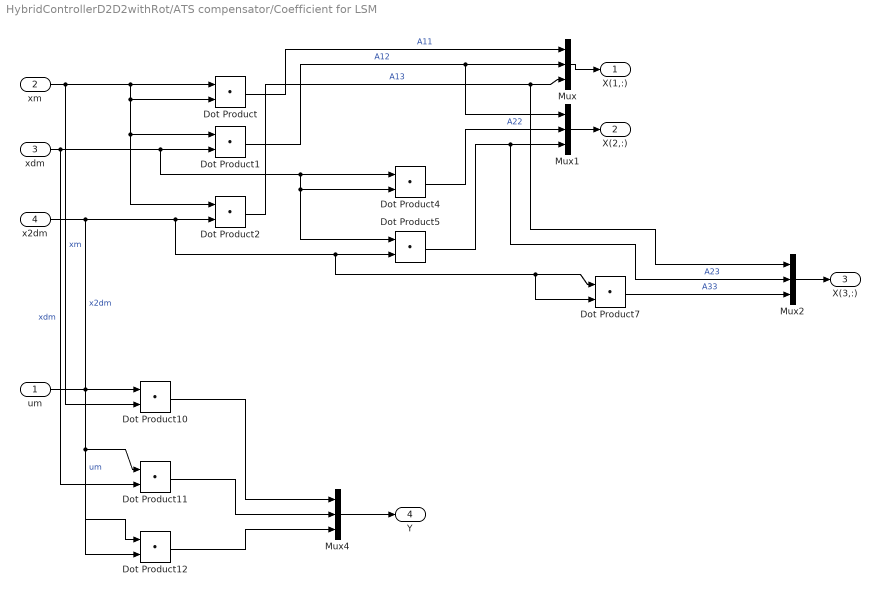
== system HybridControllerD2D2withRot/ATS compensator/Coefficient for LSM ==
  um : Inport
  xm : Inport  Port=2
  xdm : Inport  Port=3
  x2dm : Inport  Port=4
  Dot Product{,1..2,4..5,7,10..12} (9 alike) : DotProduct  InputSameDT=on  OutDataTypeStr=Inherit: Inherit via internal rule
  Mux{,1..2,4} (4 alike) : Mux  Inputs=3
  X(1,:) : Outport
  X(2,:) : Outport  Port=2
  X(3,:) : Outport  Port=3
  Y : Outport  Port=4
  wires:
  xm/1 -> Dot Product/1, Dot Product/2, Dot Product1/1, Dot Product2/1, Dot Product10/2  "xm"
  xdm/1 -> Dot Product1/2, Dot Product4/1, Dot Product4/2, Dot Product5/1, Dot Product11/2  "xdm"
  x2dm/1 -> Dot Product2/2, Dot Product5/2, Dot Product7/1, Dot Product7/2, Dot Product12/2  "x2dm"
  um/1 -> Dot Product10/1, Dot Product11/1, Dot Product12/1  "um"
  Dot Product/1 -> Mux/1  "A11"
  Dot Product1/1 -> Mux/2, Mux1/1  "A12"
  Dot Product2/1 -> Mux/3, Mux2/1  "A13"
  Mux/1 -> X(1,:)/1
  Dot Product4/1 -> Mux1/2  "A22"
  Dot Product5/1 -> Mux1/3, Mux2/2  "A23"
  Mux1/1 -> X(2,:)/1
  Dot Product7/1 -> Mux2/3  "A33"
  Mux2/1 -> X(3,:)/1
  Mux4/1 -> Y/1
  Dot Product10/1 -> Mux4/1
  Dot Product11/1 -> Mux4/2
  Dot Product12/1 -> Mux4/3

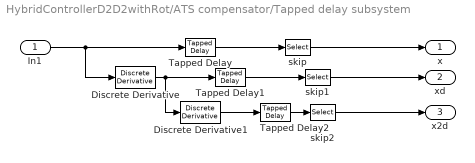
== system HybridControllerD2D2withRot/ATS compensator/Tapped delay subsystem ==
  In1 : Inport
  Discrete Derivative : simulink/Discrete/Discrete Derivative  gainval=1.0  ICPrevScaledInput=0.0  OutMin=[]  OutMax=[]  OutDataType=fixdt(1, 16)  OutScaling=2^-10  DoSatur=off
  Discrete Derivative1 : simulink/Discrete/Discrete Derivative  gainval=1.0  ICPrevScaledInput=0.0  OutMin=[]  OutMax=[]  OutDataType=fixdt(1, 16)  OutScaling=2^-10  DoSatur=off
  Tapped Delay : simulink/Discrete/Tapped Delay  vinit=0.0  samptime=-1  NumDelays=Nl  DelayOrder=Oldest  includeCurrent=off
  Tapped Delay1 : simulink/Discrete/Tapped Delay  vinit=0.0  samptime=-1  NumDelays=Nl  DelayOrder=Oldest  includeCurrent=off
  Tapped Delay2 : simulink/Discrete/Tapped Delay  vinit=0.0  samptime=-1  NumDelays=Nl  DelayOrder=Oldest  includeCurrent=off
  skip : Selector  InputPortWidth=Nl  IndexOptions=Index vector (dialog)  Indices=[1:SN:Nl]  OutputSizes=1
  skip1 : Selector  InputPortWidth=Nl  IndexOptions=Index vector (dialog)  Indices=[1:SN:Nl]  OutputSizes=1
  skip2 : Selector  InputPortWidth=Nl  IndexOptions=Index vector (dialog)  Indices=[1:SN:Nl]  OutputSizes=1
  x : Outport
  xd : Outport  Port=2
  x2d : Outport  Port=3
  wires:
  In1/1 -> Discrete Derivative/1, Tapped Delay/1
  Discrete Derivative/1 -> Discrete Derivative1/1, Tapped Delay1/1
  Discrete Derivative1/1 -> Tapped Delay2/1
  Tapped Delay/1 -> skip/1
  Tapped Delay1/1 -> skip1/1
  Tapped Delay2/1 -> skip2/1
  skip/1 -> x/1
  skip1/1 -> xd/1
  skip2/1 -> x2d/1

== system HybridControllerD2D2withRot/Filter/extract1 ==
  In1 : Inport
  Selector : Selector  InputPortWidth=size  IndexOptions=Index vector (dialog)  Indices=id  OutputSizes=1
  Out1 : Outport
  wires:
  Selector/1 -> Out1/1
  In1/1 -> Selector/1

== system HybridControllerD2D2withRot/Filter/extract2 ==
  In1 : Inport
  Selector : Selector  InputPortWidth=size  IndexOptions=Index vector (dialog)  Indices=id  OutputSizes=1
  Out1 : Outport
  wires:
  Selector/1 -> Out1/1
  In1/1 -> Selector/1

== system HybridControllerD2D2withRot/Filter/extract3 ==
  In1 : Inport
  Selector : Selector  InputPortWidth=size  IndexOptions=Index vector (dialog)  Indices=id  OutputSizes=1
  Out1 : Outport
  wires:
  Selector/1 -> Out1/1
  In1/1 -> Selector/1

== system HybridControllerD2D2withRot/Filter/extract4 ==
  In1 : Inport
  Selector : Selector  InputPortWidth=size  IndexOptions=Index vector (dialog)  Indices=id  OutputSizes=1
  Out1 : Outport
  wires:
  Selector/1 -> Out1/1
  In1/1 -> Selector/1

== system HybridControllerD2D2withRot/Filter/extract5 ==
  In1 : Inport
  Selector : Selector  InputPortWidth=size  IndexOptions=Index vector (dialog)  Indices=id  OutputSizes=1
  Out1 : Outport
  wires:
  Selector/1 -> Out1/1
  In1/1 -> Selector/1

== system HybridControllerD2D2withRot/Filter/filter2 ==
  In1 : Inport
  notch filter : Subsystem  mask(Notch Filter){freq=9, bw=7, depth=-0.8, gain=1, samplePeriod=controlPeriod}
      mask prompts: freq "Center frequency (Hz)"; bw "3 dB bandwidth (Hz)"; depth "Notch depth"; gain "DC gain"; samplePeriod "Sample period (sec)"
      mask init:
      | if (0 < freq) & (freq * samplePeriod < 0.5)
      | 	t	 = tan(pi * bw * samplePeriod);	
      | 	k1	 = -cos(2 * pi * freq * samplePeriod);
      | 	k1	 = max(min(k1, 1), -1);
      | 	k2	 = (1.0 - t) / (1.0 + t);
      | 	k2	 = max(min(k2, 1), -1);
      | 	w0	 =  gain + 0.5 * depth;
      | 	w1	 = -0.5 * depth;
      | else
      | 	k1	 = 0.0;
      | 	k2	 = 0.0;
      | 	w0	 = gain;
      | 	w1	 = 0.0;
      | end
      | a1	= k1 * (1 + k2);
      | a2	= k2;
      | b	= [w0+w1*a2 (w0+w1)*a1 w1+w0*a2];
      | a	= [1 a1 a2];
  notch filter1 : Subsystem  mask(Notch Filter){freq=30, bw=8, depth=-0.8, gain=1, samplePeriod=controlPeriod}
      mask prompts: freq "Center frequency (Hz)"; bw "3 dB bandwidth (Hz)"; depth "Notch depth"; gain "DC gain"; samplePeriod "Sample period (sec)"
      mask init: same as HybridControllerD2D2withRot/Filter/filter2/notch filter
  notch filter2 : Subsystem  mask(Notch Filter){freq=33, bw=8, depth=-0.8, gain=1, samplePeriod=controlPeriod}
      mask prompts: freq "Center frequency (Hz)"; bw "3 dB bandwidth (Hz)"; depth "Notch depth"; gain "DC gain"; samplePeriod "Sample period (sec)"
      mask init: same as HybridControllerD2D2withRot/Filter/filter2/notch filter
  Out1 : Outport
  wires:
  notch filter/1(out) -> notch filter1/1(inp)
  In1/1 -> notch filter/1(inp)
  notch filter1/1(out) -> notch filter2/1(inp)
  notch filter2/1(out) -> Out1/1

== system HybridControllerD2D2withRot/LoadCells/extract1 ==
  In1 : Inport
  Selector : Selector  InputPortWidth=size  IndexOptions=Index vector (dialog)  Indices=id  OutputSizes=1
  Out1 : Outport
  wires:
  Selector/1 -> Out1/1
  In1/1 -> Selector/1

== system HybridControllerD2D2withRot/LoadCells/extract2 ==
  In1 : Inport
  Selector : Selector  InputPortWidth=size  IndexOptions=Index vector (dialog)  Indices=id  OutputSizes=1
  Out1 : Outport
  wires:
  Selector/1 -> Out1/1
  In1/1 -> Selector/1

== system HybridControllerD2D2withRot/LoadCells/extract3 ==
  In1 : Inport
  Selector : Selector  InputPortWidth=size  IndexOptions=Index vector (dialog)  Indices=id  OutputSizes=1
  Out1 : Outport
  wires:
  Selector/1 -> Out1/1
  In1/1 -> Selector/1

== system HybridControllerD2D2withRot/LoadCells/extract4 ==
  In1 : Inport
  Selector : Selector  InputPortWidth=size  IndexOptions=Index vector (dialog)  Indices=id  OutputSizes=1
  Out1 : Outport
  wires:
  Selector/1 -> Out1/1
  In1/1 -> Selector/1

== system HybridControllerD2D2withRot/LoadCells/extract5 ==
  In1 : Inport
  Selector : Selector  InputPortWidth=size  IndexOptions=Index vector (dialog)  Indices=id  OutputSizes=1
  Out1 : Outport
  wires:
  Selector/1 -> Out1/1
  In1/1 -> Selector/1

== system HybridControllerD2D2withRot/LoadCells/filter2 ==
  In1 : Inport
  notch filter : Subsystem  mask(Notch Filter){freq=9, bw=7, depth=-0.8, gain=1, samplePeriod=controlPeriod}
      mask prompts: freq "Center frequency (Hz)"; bw "3 dB bandwidth (Hz)"; depth "Notch depth"; gain "DC gain"; samplePeriod "Sample period (sec)"
      mask init: same as HybridControllerD2D2withRot/Filter/filter2/notch filter
  notch filter1 : Subsystem  mask(Notch Filter){freq=30, bw=8, depth=-0.8, gain=1, samplePeriod=controlPeriod}
      mask prompts: freq "Center frequency (Hz)"; bw "3 dB bandwidth (Hz)"; depth "Notch depth"; gain "DC gain"; samplePeriod "Sample period (sec)"
      mask init: same as HybridControllerD2D2withRot/Filter/filter2/notch filter
  notch filter2 : Subsystem  mask(Notch Filter){freq=33, bw=8, depth=-0.8, gain=1, samplePeriod=controlPeriod}
      mask prompts: freq "Center frequency (Hz)"; bw "3 dB bandwidth (Hz)"; depth "Notch depth"; gain "DC gain"; samplePeriod "Sample period (sec)"
      mask init: same as HybridControllerD2D2withRot/Filter/filter2/notch filter
  Out1 : Outport
  wires:
  notch filter/1(out) -> notch filter1/1(inp)
  In1/1 -> notch filter/1(inp)
  notch filter1/1(out) -> notch filter2/1(inp)
  notch filter2/1(out) -> Out1/1

== system HybridControllerD2D2withRot/Offset/If Action ==
  In1 : Inport
  Action Port : ActionPort  PropagateVarSize=During execution  ActionType=then
  Data Store Read : DataStoreRead  DataStoreName=x0  SampleTime=controlPeriod
  Data Store Write : DataStoreWrite  DataStoreName=x0
  Gain : Gain  Gain=1/nOffset  SaturateOnIntegerOverflow=on  OutDataTypeStr=Inherit: Same as input  ParamDataTypeStr=Inherit: Same as input
  Sum : Sum  Inputs=|++  SaturateOnIntegerOverflow=on  InputSameDT=on  OutDataTypeStr=Inherit: Same as first input
  wires:
  Data Store Read/1 -> Sum/2
  Sum/1 -> Data Store Write/1
  Gain/1 -> Sum/1
  In1/1 -> Gain/1

== system HybridControllerD2D2withRot/xPC HC/Offset ==
  In1 : Inport
  Constant : Constant  Value=zeros(1,nS)
  Counter : simulink/Sources/Counter Free-Running  NumBits=32  tsamp=-1
  Data Store Memory : DataStoreMemory  DataStoreName=x0  InitialValue=zeros(1,nS)  OutDataTypeStr=double
  Data Store Read : DataStoreRead  DataStoreName=x0
  If : If  IfExpression=u1 < nOffset  ShowElse=off
  If Action : Subsystem  TreatAsAtomicUnit=on
  Sum1 : Sum  Inputs=+-|  SaturateOnIntegerOverflow=on  InputSameDT=on  OutDataTypeStr=Inherit: Same as first input
  Switch : Switch  Threshold=nOffset  SaturateOnIntegerOverflow=on  InputSameDT=on
  Out1 : Outport
  wires:
  Switch/1 -> Out1/1
  Sum1/1 -> Switch/1
  Data Store Read/1 -> Sum1/2
  In1/1 -> If Action/1(In1), Sum1/1
  Constant/1 -> Switch/3
  Counter/1 -> Switch/2, If/1
  If/1 -> If Action/Action

== system HybridControllerD2D2withRot/xPC HC/Offset1 ==
  In1 : Inport
  Constant : Constant  Value=zeros(1,nS)
  Counter : simulink/Sources/Counter Free-Running  NumBits=32  tsamp=-1
  Data Store Memory : DataStoreMemory  DataStoreName=x0  InitialValue=zeros(1,nS)  OutDataTypeStr=double
  Data Store Read : DataStoreRead  DataStoreName=x0
  If : If  IfExpression=u1 < nOffset  ShowElse=off
  If Action : Subsystem  TreatAsAtomicUnit=on
  Sum1 : Sum  Inputs=+-|  SaturateOnIntegerOverflow=on  InputSameDT=on  OutDataTypeStr=Inherit: Same as first input
  Switch : Switch  Threshold=nOffset  SaturateOnIntegerOverflow=on  InputSameDT=on
  Out1 : Outport
  wires:
  Switch/1 -> Out1/1
  Sum1/1 -> Switch/1
  Data Store Read/1 -> Sum1/2
  In1/1 -> If Action/1(In1), Sum1/1
  Constant/1 -> Switch/3
  Counter/1 -> Switch/2, If/1
  If/1 -> If Action/Action

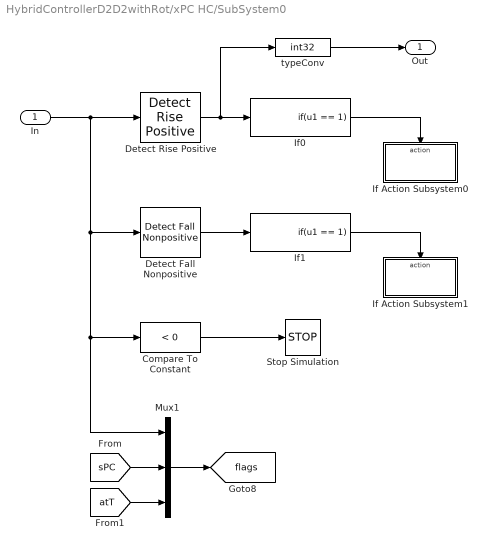
== system HybridControllerD2D2withRot/xPC HC/SubSystem0 ==
  In : Inport
  Compare To Constant : simulink/Logic and Bit Operations/Compare To Constant  relop=<  const=0  OutDataTypeStr=boolean
  Detect Fall Nonpositive : simulink/Logic and Bit Operations/Detect Fall Nonpositive  vinit=0  OutDataTypeStr=uint8
  Detect Rise Positive : simulink/Logic and Bit Operations/Detect Rise Positive  vinit=0  OutDataTypeStr=uint8
  If Action Subsystem0 : Subsystem  TreatAsAtomicUnit=on
  If Action Subsystem1 : Subsystem  TreatAsAtomicUnit=on
  If0 : If  IfExpression=u1 == 1  ShowElse=off
  If1 : If  IfExpression=u1 == 1  ShowElse=off
  Mux1 : Mux  Inputs=3
  Stop Simulation : Stop
  typeConv : DataTypeConversion  OutDataTypeStr=int32  SaturateOnIntegerOverflow=on  RndMeth=Zero
  Out : Outport
  tag scope: flags=global
  wires:
  Detect Rise Positive/1 -> If0/1, typeConv/1
  Detect Fall Nonpositive/1 -> If1/1
  If1/1 -> If Action Subsystem1/Action
  If0/1 -> If Action Subsystem0/Action
  typeConv/1 -> Out/1
  Mux1/1 -> [flags]
  [sPC] -> Mux1/2
  [atT] -> Mux1/3
  In/1 -> Detect Rise Positive/1, Detect Fall Nonpositive/1, Compare To Constant/1, Mux1/1
  Compare To Constant/1 -> Stop Simulation/1

== system HybridControllerD2D2withRot/xPC HC/SubSystem1 ==
  measDsp : Inport
  measFrc : Inport  Port=2
  Constant : Constant  Value=iDelay
  For Each Subsystem : Subsystem  TreatAsAtomicUnit=on
  Gain4 : Gain  SaturateOnIntegerOverflow=on  OutDataTypeStr=Inherit: Same as input  ParamDataTypeStr=Inherit: Same as input
  Mux : Mux  Inputs=2
  SubSystem2 : Subsystem  TreatAsAtomicUnit=on
  Subsystem2 : Subsystem
  measSig : Outport
  tag scope: measDsp=global, measFrc=global
  wires:
  Subsystem2/1(trig) -> SubSystem2/Trigger
  [counter] -> Subsystem2/1(i), For Each Subsystem/1(i)
  Gain4/1 -> measSig/1
  Constant/1 -> For Each Subsystem/2(iDelay)
  measDsp/1 -> [measDsp], For Each Subsystem/3(measDsp)
  measFrc/1 -> For Each Subsystem/4(measFrc), [measFrc]
  For Each Subsystem/1(measDspOut) -> Mux/1
  For Each Subsystem/2(measFrcOut) -> Mux/2
  Mux/1 -> Gain4/1
